simulink model "AM_envelope_2023b"  (R2023b)
settings: Solver=ode45  StartTime=0.0  StopTime=10  RelTol=1e-3  EnableMultiTasking=on
libraries: dspfdesign x1
settings Model: Creator=morelos_zaragoza  LastModifiedBy=14083
settings SolverCC: AlgebraicLoopSolver=TrustRegion
settings DataIOCC: LimitDataPoints=on  SaveFormat=Array  SignalLoggingSaveFormat=ModelDataLogs  ReturnWorkspaceOutputs=off
settings OptimizationCC: ExpressionDepthLimit=2147483647  InitFltsAndDblsToZero=on  LifeSpan=inf
settings DebuggingCC: SaveWithParameterizedLinksMsg=none  UnderspecifiedInitializationDetection=Classic  MergeDetectMultiDrivingBlocksExec=none  SignalResolutionControl=TryResolveAllWithWarning  SolverPrmCheckMsg=warning  MultiTaskDSMMsg=warning  MultiTaskCondExecSysMsg=none  FcnCallInpInsideContextMsg=warning  UnconnectedInputMsg=warning  UnconnectedOutputMsg=warning  UnconnectedLineMsg=warning  StateNameClashWarn=warning  SFUnexpectedBacktrackingDiag=warning  SFNoUnconditionalDefaultTransitionDiag=warning  SFExecutionAtInitializationDiag=none  ArithmeticOperatorsInVariantConditions=warning
settings HardwareCC: ProdBitPerPointer=32  ProdBitPerSizeT=32  ProdBitPerPtrDiffT=32  ProdLargestAtomicFloat=None  ProdIntDivRoundTo=Undefined  ProdEndianess=Unspecified  ProdWordSize=32  ProdHWDeviceType=32-bit Generic
settings ModelReferenceCC: PropagateSignalLabelsOutOfModel=off
settings SFSimCC: SimUseLocalCustomCode=off  CustomCodeUndefinedFunction=UseInterfaceOnly
settings RTWCC: RTWUseLocalCustomCode=off
settings CodeAppCC: StateflowObjectComments=on
settings GRTTargetCC: TargetFcnLib=ansi_tfl_tmw.mat  TargetLangStandard=C89/C90 (ANSI)  CombineOutputUpdateFcns=off  GRTInterface=on
settings ConfigComp: CovMetricSettings=dw  CovSaveCumulativeToWorkspaceVar=on  CovSaveSingleToWorkspaceVar=on  CovExternalEMLEnable=off

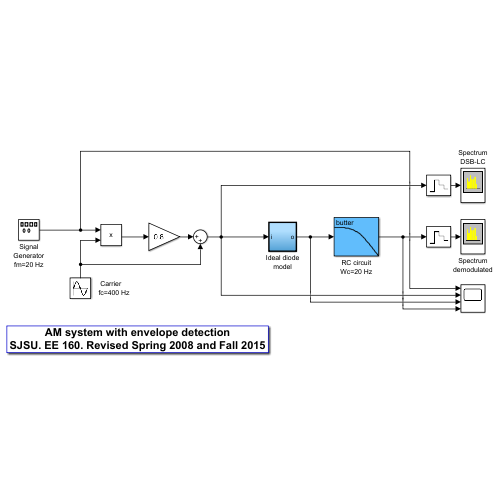
[thumbnail: Simulink's stored preview of the top-level diagram]
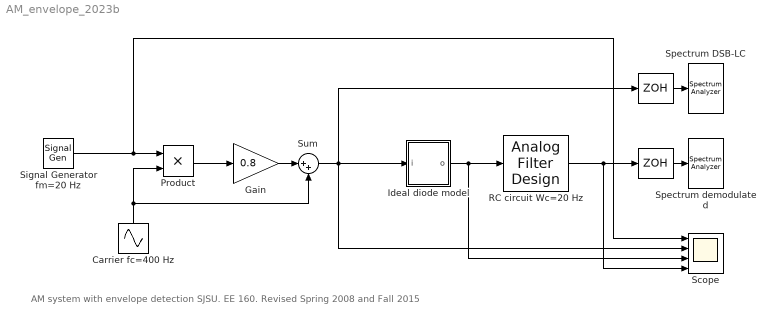
== system AM_envelope_2023b ==
  note: AM system with envelope detection
      | SJSU. EE 160. Revised Spring 2008 and Fall 2015
  "  " : ZeroOrderHold  SampleTime=1/(25*90)
  "   " : ZeroOrderHold  SampleTime=1/(25*90)
  "   Carrier fc=400 Hz" : Sin  Frequency=2*pi*400  SampleTime=0
  Gain : Gain  Gain=0.8
  Ideal diode model : Subsystem  TreatAsAtomicUnit=on
  Product : Product  RndMeth=Zero
  RC circuit Wc=20 Hz : dspfdesign/Analog Filter Design  method=Butterworth  filttype=Lowpass  N=1  Wlo=2*pi*20  Whi=2*pi*110  Rp=2  Rs=60
  Scope : Scope  NumInputPorts=4
  Signal Generator fm=20 Hz : SignalGenerator  Frequency=10
  Spectrum DSB-LC : SpectrumAnalyzer  WindowPosition=[937.000000,475.000000,581.000000,357.000000,]  Visible=on  ScopeFrameLocation=window  AxesScaling=Manual  FFTLength=2048  YLabel=Magnitude  YLimits=[-30.16578143,33.35616328]
  Spectrum demodulated : SpectrumAnalyzer  WindowPosition=[936.000000,32.000000,586.000000,412.000000,]  Visible=on  ScopeFrameLocation=window  AxesScaling=Manual  FFTLength=2048  YLabel=Magnitude  YLimits=[-40.82959398,36.29177125]
  Sum : Sum  Inputs=|++
  wires:
  Signal Generator fm=20 Hz/1 -> Product/1, Scope/1
  "   Carrier fc=400 Hz"/1 -> Product/2, Sum/2
  "  "/1 -> Spectrum DSB-LC/1
  "   "/1 -> Spectrum demodulated/1
  RC circuit Wc=20 Hz/1 -> "   "/1, Scope/4
  Ideal diode model/1(o) -> RC circuit Wc=20 Hz/1, Scope/3
  Gain/1 -> Sum/1
  Product/1 -> Gain/1
  Sum/1 -> Ideal diode model/1(i), "  "/1, Scope/2

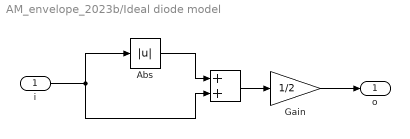
== system AM_envelope_2023b/Ideal diode model ==
  i : Inport
  " " : Sum
  Abs : Abs  SaturateOnIntegerOverflow=off
  Gain : Gain  Gain=1/2
  o : Outport
  wires:
  i/1 -> Abs/1, " "/2
  Abs/1 -> " "/1
  " "/1 -> Gain/1
  Gain/1 -> o/1
